simulink model "Lab_3_2"  (R2023a)
settings: Solver=VariableStepAuto  StartTime=0.0  StopTime=10.0  RelTol=1e-3
libraries: dspfdesign x2
settings Model: Creator=mluser  LastModifiedBy=mluser
settings OptimizationCC: ReuseModelBlockBuffer=off

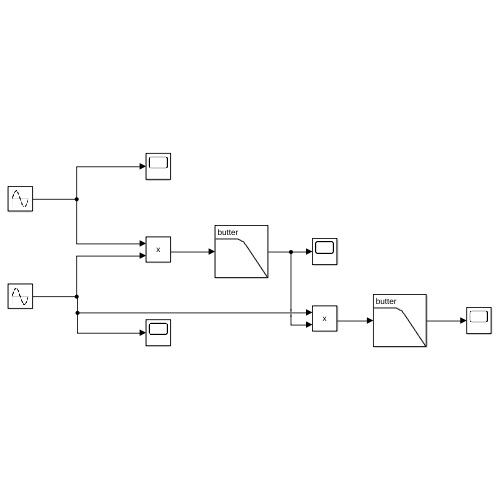
[thumbnail: Simulink's stored preview of the top-level diagram]
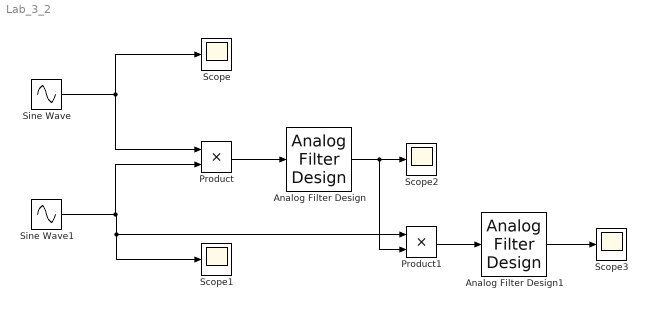
== system Lab_3_2 ==
  Analog Filter Design : dspfdesign/Analog Filter Design  method=Butterworth  filttype=Lowpass  N=3  Wlo=4  Whi=80  Rp=2  Rs=40
  Analog Filter Design1 : dspfdesign/Analog Filter Design  method=Butterworth  filttype=Lowpass  N=3  Wlo=4  Whi=80  Rp=2  Rs=40
  Product : Product
  Product1 : Product
  Scope{,1..3} (4 alike) : Scope
  Sine Wave : Sin  Amplitude=5  SampleTime=0
  Sine Wave1 : Sin  Amplitude=5  Frequency=10  SampleTime=0
  wires:
  Sine Wave/1 -> Product/1, Scope/1
  Sine Wave1/1 -> Product/2, Product1/1, Scope1/1
  Product/1 -> Analog Filter Design/1
  Analog Filter Design/1 -> Scope2/1, Product1/2
  Product1/1 -> Analog Filter Design1/1
  Analog Filter Design1/1 -> Scope3/1
